simulink model "Punto3"  (R2018b)
settings: Solver=VariableStepAuto  StartTime=0.0  StopTime=15.0  RelTol=1e-3
libraries: simulink x1
settings Model: Creator=MichhaPC  LastModifiedBy=MichhaPC

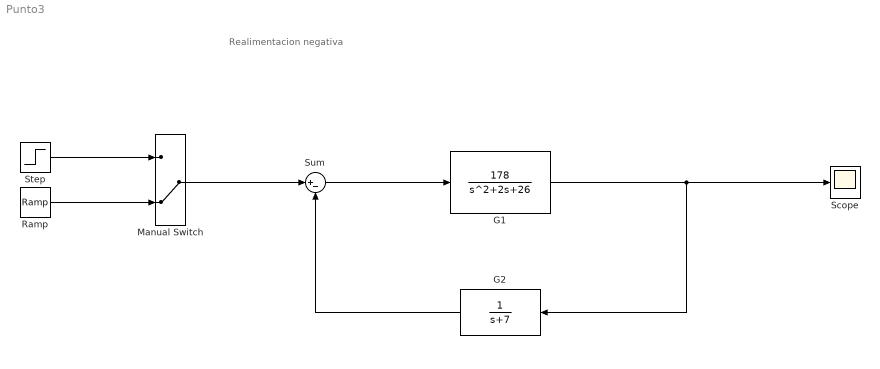
== system Punto3 ==
  note: Realimentacion negativa
  G1 : TransferFcn  Numerator=[178]  Denominator=[1 2 26]
  G2 : TransferFcn  Denominator=[1 7]
  Manual Switch : ManualSwitch  CurrentSetting=0
  Ramp : simulink/Sources/Ramp  slope=0.1  start=0  InitialOutput=0
  Scope : Scope
  Step : Step  Time=0.1  SampleTime=0
  Sum : Sum  Inputs=|+-
  wires:
  Sum/1 -> G1/1
  G1/1 -> G2/1, Scope/1
  G2/1 -> Sum/2
  Manual Switch/1 -> Sum/1
  Step/1 -> Manual Switch/1
  Ramp/1 -> Manual Switch/2
